simulink model "IARC_Nonlinear_Sensors"  (R2018a)
settings: Solver=ode1  StartTime=0.0  StopTime=20  FixedStep=T  RelTol=1e-3  EnableMultiTasking=on
undefined symbols (not defined in the file): A_1df, A_2df, alpha3, alpha_rp, alpha_x, alpha_z, an1, an1_v, an2, an3, bn1, bn1_v, bn2, bn3, dc_M_x, delta3, Epsilon3, F, g, Gamma1, Gamma2, Gamma3, Gamma4, gamma4_0, gamma_d_x, gamma_rp_0, gamma_x_0, gamma_z_0, Gammax, I, I_add, I_add_time, Jx, Jy, Jyaw, K, k1, k10, k11, k12, k2, k3, k4, k5, k6, k7, k8, k9, Ky, L, Light, LIMIT_CMD_PITCH, LIMIT_CMD_ROLL, LIMIT_CMD_xy, LIMIT_uCMD_HEIGHT, m, m_add, m_add_time, magnitude, MIL ... (+67)
libraries: simulink x131, simulink_extras x5, UAV_Control x4, aerolibwind2 x1
(part 3 of 6)

== system IARC_Nonlinear_Sensors/ARC Controller/Attitutde Control/Yaw control/e12 ==
  Add : Sum
  Discrete Derivative2 : simulink/Discrete/Discrete Derivative  gainval=1.0  ICPrevScaledInput=0.0  OutMin=[]  OutMax=[]  OutDataType=fixdt(1, 16)  OutScaling=2^-10  DoSatur=off
  Sum1 : Sum  Inputs=-+|
  Sum3 : Sum  Inputs=|+-
  Transfer Fcn3 : TransferFcn  Denominator=A_1df
  k11 : Gain  Gain=k11
  e12 : Outport
  wires:
  [psi_des] -> Sum3/2, Discrete Derivative2/1
  [psi] -> Sum3/1
  Sum1/1 -> Add/2  "ev"
  Sum3/1 -> k11/1  "ex"
  Add/1 -> e12/1
  [psi_dot] -> Sum1/2
  Discrete Derivative2/1 -> Transfer Fcn3/1
  k11/1 -> Add/1
  Transfer Fcn3/1 -> Sum1/1

== system IARC_Nonlinear_Sensors/ARC Controller/Attitutde Control/Yaw control/f ==
  " " : Trigonometry  Operator=sincos
  "  " : Trigonometry
  "      " : Trigonometry  Operator=cos
  Add : Sum  Inputs=++-
  Add1 : Sum  Inputs=+-
  Constant1 : Constant  Value=(Jy-Jyaw)/Jx
  Discrete Derivative1 : simulink/Discrete/Discrete Derivative  gainval=1.0  ICPrevScaledInput=0.0  OutMin=[]  OutMax=[]  OutDataType=fixdt(1, 16)  OutScaling=2^-10  DoSatur=off
  Discrete Derivative2 : simulink/Discrete/Discrete Derivative  gainval=1.0  ICPrevScaledInput=0.0  OutMin=[]  OutMax=[]  OutDataType=fixdt(1, 16)  OutScaling=2^-10  DoSatur=off
  Discrete Derivative3 : simulink/Discrete/Discrete Derivative  gainval=1.0  ICPrevScaledInput=0.0  OutMin=[]  OutMax=[]  OutDataType=fixdt(1, 16)  OutScaling=2^-10  DoSatur=off
  Ground : Ground
  Product1 : Product
  Product2 : Product  Inputs=**/
  Product4 : Product  Inputs=***/
  Selector1 : Selector  InputPortWidth=3  IndexOptions=Index vector (dialog)  Indices=[2 3]  OutputSizes=1
  q.r : Product  Inputs=*
  Out1 : Outport
  wires:
  [phi] -> "      "/1
  "      "/1 -> Product4/4
  Product4/1 -> Add/2
  q.r/1 -> Product4/2
  Selector1/1 -> q.r/1
  [pqr_est] -> Selector1/1
  Constant1/1 -> Product4/1
  Discrete Derivative1/1 -> Product2/1
  " "/2 -> Product2/3
  Add1/1 -> Product2/2
  Product1/1 -> Add1/2
  " "/1 -> Product1/2
  Discrete Derivative2/1 -> Product1/1
  Discrete Derivative3/1 -> Add1/1
  [phi] -> " "/1, Discrete Derivative1/1
  Add/1 -> Out1/1
  Product2/1 -> Add/1
  [theta] -> "  "/1
  "  "/1 -> Product4/3
  [psi] -> Discrete Derivative2/1
  [theta] -> Discrete Derivative3/1
  Ground/1 -> Add/3

== system IARC_Nonlinear_Sensors/ARC Controller/Attitutde Control/Yaw control/f(x) ==
  Add : Sum  Inputs=+--
  Discrete Derivative1 : simulink/Discrete/Discrete Derivative  gainval=1.0  ICPrevScaledInput=0.0  OutMin=[]  OutMax=[]  OutDataType=fixdt(1, 16)  OutScaling=2^-10  DoSatur=off
  T1 .. : Subsystem
  f : Subsystem
  Out1 : Outport
  wires:
  [psi_dot] -> Discrete Derivative1/1
  Discrete Derivative1/1 -> Add/1
  Add/1 -> Out1/1
  f/1(Out1) -> Add/2
  T1 ../1(Out1) -> Add/3

== system IARC_Nonlinear_Sensors/ARC Controller/Attitutde Control/Yaw control/phi ==
  "  " : Trigonometry  Operator=cos
  "   " : Trigonometry  Operator=cos
  Constant : Constant
  Gain10 : Gain  Gain=1/Ky
  Mux : Mux  Inputs=2
  Notch Filter2 : Subsystem
  Product2 : Product  Inputs=*/*
  rotor : TransferFcn  Numerator=1  Denominator=[Tm 1]
  Out1 : Outport
  wires:
  Mux/1 -> Out1/1
  Constant/1 -> Mux/2
  Notch Filter2/1(p) -> rotor/1
  [T3] -> Gain10/1
  "  "/1 -> Product2/1
  "   "/1 -> Product2/2
  rotor/1 -> Product2/3
  Product2/1 -> Mux/1
  [theta] -> "  "/1
  [phi] -> "   "/1
  Gain10/1 -> Notch Filter2/1(u)

== system IARC_Nonlinear_Sensors/ARC Controller/Attitutde Control/pitch control/Adaptation Law_X ==
  Phi_D : Inport
  error : Inport  Port=2
  f(x) : Inport  Port=3
  Phi_I : Inport  Port=4
  Adapt : Inport  Port=5
  " " : Subsystem
  Constant2 : Constant  Value=theta1_Max(1,2)
  Constant5 : Constant  Value=theta1_Max(1,1)
  Constant6 : Constant  Value=theta1_Min(1,2)
  Constant8 : Constant  Value=theta1_Min(1,1)
  Demux1 : Demux  Outputs=2
  Demux2 : Demux  Outputs=2
  Gain3 : Gain  Gain=K*L
  "IARC, Physical Model Based Parameter Estimation (69)_pitch (theta)" : Subsystem  AncestorBlock=|  mask(Physical Model Based Parameter Estimation){mu1=mu1_rp, mu2=mu2_rp, alpha=alpha_rp, nu=nu_rp, gamma0=gamma_rp_0, Rho_M=Rho_M_rp, Rho_L=Rho_L_rp, v=v_rp, theta_0=theta2_0, theta_max=theta2_Max, theta_min=theta2_Min, Theta_dot_M=theta_dot_M_rp, Tau=Tau_rp, t0=t0, Norm_ON=on}
      | UAV_Control/IARC, Physical Model Based 
      | Parameter Estimation (69)
      mask prompts: mu1 "forgetting factor, mu1:"; mu2 "RLS parameter, mu2:"; alpha "forgetting factor, alpha:"; nu "normalizing factor, nu:"; gamma0 "Initial adaptation gain:"; Rho_M "Upper bound for the adaptation gain:"; Rho_L "Lower bound for the adaptation gain:"; v "Eigenvector of Gamma_max:"; Theta_dot_M "Theta dot max:"; Tau "Filter time constant:"; t0 "Initialization Delay:"; Norm_ON "Use Normalized formula"
      mask Help:
      | Filtered system dynamics:
      | H_f (s)  is any stable LTI filter transfer function
      | x_f=H_f [x]
      | φ_f=H_f [φ(x)]
      | u_f=H_f [u]
      | 
      | y_p=x ̇_f−u_f
      | y ̂_p=φ_f^T θ ̂
      | Prediction error:
      | ϵ=y_p−y ̂_p
      | 
      | recursive estimation algorithms, the generalized parameter estimation algorithm (PAA) with covariance limiting:
      | 
      | θ ̂  ̇(t)=Γ(t) φ_f (t)ϵ(t)
      | D_Γ=μ_1 (t)Γ(t)−μ_2 (t)Γ(t) φ_f (t) φ_f (t)^T Γ(t)
      | Γ ̇(t)=D_Γ, if λ_M (Γ(t))<ρ_M  or v_M^T D_Γ v_M<0 )
      |          0        else
      | 
      | μ_1  and μ_2  are two non-negative functions
      | ρ_M  is a preset upper bound for the covariance matrix Γ(t)
      | μ_1  represents the forgetting factor (μ_1=0 for not forgetting)
      | μ_2: 1 stands for the standard least squares type estimation algorithm
      |        0 stands for  the gradient type estimation algorithm
      |        range: 0≤μ_2<2
      | Initialization of the covariance matrix: Γ(0)<ρ_M I_p
      | 
      | IARC designs completely separate the parameter estimation law design from the underlying robust control law to give better parameter estimates than possible with DARC designs. In addition, explicit on-line signal excitation level monitoring can be employed to significantly improve the accuracy of  parameter estimates.
      | 
      | Normalized Method:
      | θ ̂  ̇(t)=(Γ(t) φ_f (t)ϵ(t))/(1+νφ_f^T Γφ_f )
      | D_Γ=αΓ(t)−(Γ(t) φ_f (t) φ_f (t)^T Γ(t))/(1+νφ_f^T Γφ_f )
      | Γ ̇(t)=D_Γ, if λ_M (Γ(t))<ρ_M  or v_M^T D_Γ v_M<0
      |           0       else
      mask Display:
      | port_label('input',1,'f(x)','texmode','on')
      | port_label('input',2,'\phi','texmode','on')
      | port_label('input',3,'Adapt','texmode','on')
      | 
      | port_label('output',1,'\theta_{hat}','texmode','on')
  Integral Type Adaptation Law Discontinuous Projection1 : Subsystem  AncestorBlock=|  mask(IntegralTypeAdaptationLaw){theta=theta1, theta0=theta1_0, theta_max=theta1_Max, theta_min=theta1_Min, gamma=Gamma1, t0=t0, Adaptation_ON=on}
      | UAV_Control/Integral Type
      | Adaptation Law
      | Discontinuous Projection
      mask prompts: theta "Actual value of theta:"; theta0 "Initial value of theta:"; theta_max "Maximum value of theta:"; theta_min "Minimum value of theta:"; gamma "Adaptation Rate:"; t0 "Initialization Delay:"; Adaptation_ON "Activate adaptation:"
      mask help: Applies an Integral-type adaptation law with discontinuous projection on the parameter theta.
      mask Help:
      | Applies an Integral-type adaptation law with discontinuous projection on the parameter theta.
      | 
      | theta_est_dot=Gamma*Phi*e
      | theta=proj( int(theta_estdot) )
      | 
      | theta_min < theta_est <  theta_max
      | 
      | Parameters:
      | 
      | Gamma: nxn diagonal matrix, adaptaion rate.
      | theta_min: nx1 vector, minimum value of the estimated vector.
      | theta_max: nx1 vector, maximum value of the estimated vector.
      | theta0: nx1 vector, initial value of the estimated vector.
      | theta: nx1 vector, actual value of the estimated vector.
      | Adaptation_On: controls the use of the adaptation law (1: active, 0: inactive)
      | 
      | Inputs:
      | Phi: regressor vector, theta0, nx1.
      | e: state error, scalar.
      | 
      | Outputs:
      | theta_est: estimated value of the parameters vector.
      mask Display:
      | port_label('input',1,'\phi','texmode','on')
      | port_label('input',2,'e','texmode','on')
      | port_label('output',1,'\theta_{hat}','texmode','on')
  J : Subsystem
  Jyy : Scope
  KL/Jyy : Scope
  Manual Switch : ManualSwitch  CurrentSetting=0
  Manual Switch1 : ManualSwitch  CurrentSetting=0
  Math Function1 : Math  Operator=reciprocal  SaturateOnIntegerOverflow=on
  Mux1 : Mux  Inputs=5
  Mux6 : Mux  Inputs=5
  Subsystem1 : Subsystem
  To File : ToFile  Commented=on  Filename=IARC21.mat  MatrixName=IARC21  SaveFormat=Timeseries
  To File1 : ToFile  Commented=on  Filename=IARC22.mat  MatrixName=IARC22  SaveFormat=Timeseries
  To Workspace1 : ToWorkspace  Commented=on  VariableName=theta11  SaveFormat=Timeseries  SampleTime=-1
  To Workspace2 : ToWorkspace  Commented=on  VariableName=theta12  SaveFormat=Timeseries  SampleTime=-1
  d1 (N.m) : Scope
  theta1 : Outport
  theta2 : Outport  Port=2
  wires:
  " "/1(Out1) -> Mux6/3  "True"
  Gain3/1 -> To File/1, Jyy/1
  Constant2/1 -> Mux6/4
  Math Function1/1 -> Gain3/1
  Demux1/1 -> Manual Switch/2, KL/Jyy/1, Mux1/2
  Mux1/1 -> Math Function1/1
  Constant6/1 -> Mux6/5
  "IARC, Physical Model Based Parameter Estimation (69)_pitch (theta)"/1(Theta_hat) -> Demux1/1
  Demux2/1 -> Mux1/1, Manual Switch/1
  error/1 -> Integral Type Adaptation Law Discontinuous Projection1/2(error)
  Integral Type Adaptation Law Discontinuous Projection1/1(theta_est) -> Demux2/1
  Manual Switch1/1 -> To Workspace2/1, theta2/1
  J/1(Out1) -> Mux1/3
  Constant8/1 -> Mux1/5
  Phi_I/1 -> "IARC, Physical Model Based Parameter Estimation (69)_pitch (theta)"/2(Phi)
  f(x)/1 -> "IARC, Physical Model Based Parameter Estimation (69)_pitch (theta)"/1(f(x))
  Constant5/1 -> Mux1/4
  Manual Switch/1 -> To Workspace1/1, theta1/1
  Phi_D/1 -> Integral Type Adaptation Law Discontinuous Projection1/1(Phi)
  Mux6/1 -> Subsystem1/1(u)
  Demux2/2 -> Mux6/1, Manual Switch1/1
  Demux1/2 -> Mux6/2, Manual Switch1/2
  Subsystem1/1(y) -> To File1/1, d1 (N.m)/1
  Adapt/1 -> "IARC, Physical Model Based Parameter Estimation (69)_pitch (theta)"/3(Adapt)

== system IARC_Nonlinear_Sensors/ARC Controller/Attitutde Control/pitch control/Ix ==
  Constant : Constant
  Gain1 : Gain  Gain=L*K
  Product1 : Product  Inputs=*/
  " " : Outport
  wires:
  [theta11_est] -> Product1/2
  Gain1/1 -> " "/1
  Product1/1 -> Gain1/1
  Constant/1 -> Product1/1

== system IARC_Nonlinear_Sensors/ARC Controller/Attitutde Control/pitch control/Phi3 ==
  Constant : Constant
  Mux1 : Mux  Inputs=2
  Product1 : Product  Inputs=*/
  alpha 4 dot : Subsystem
  Out1 : Outport
  wires:
  Mux1/1 -> Out1/1
  Product1/1 -> Mux1/1
  Constant/1 -> Mux1/2
  alpha 4 dot/1(alpha_4_dot) -> Product1/1
  [theta11_est] -> Product1/2

== system IARC_Nonlinear_Sensors/ARC Controller/Attitutde Control/pitch control/Robust term ==
  e : Inport
  phi : Inport  Port=2
  Add : Sum
  Constant3 : Constant  Value=theta_max-theta_min
  Constant6 : Constant  Value=delta
  Gain : Gain  Gain=1/(4*epsilon)
  Math Function : Math  Operator=magnitude^2  SaturateOnIntegerOverflow=on
  Math Function1 : Math  Operator=magnitude^2  SaturateOnIntegerOverflow=on
  Math Function3 : Math  Operator=magnitude^2  SaturateOnIntegerOverflow=on
  Math Function5 : Math  Operator=transpose  SaturateOnIntegerOverflow=on
  Product : Product  Multiplication=Matrix(*)
  Product1 : Product
  alpha : Outport
  wires:
  phi/1 -> Math Function1/1
  e/1 -> Gain/1
  Math Function5/1 -> Product/1
  Product1/1 -> alpha/1
  Constant3/1 -> Math Function/1
  Math Function1/1 -> Math Function5/1
  Product/1 -> Add/1
  Math Function3/1 -> Add/2
  Constant6/1 -> Math Function3/1
  Math Function/1 -> Product/2
  Add/1 -> Product1/1
  Gain/1 -> Product1/2

== system IARC_Nonlinear_Sensors/ARC Controller/Attitutde Control/pitch control/T1 .. T2 .. ==
  "  " : Trigonometry  Operator=tan
  "    " : Trigonometry
  "     " : Trigonometry  Operator=cos
  "  2" : Trigonometry  Operator=tan
  Add : Sum  Inputs=+-
  Constant : Constant  Value=Jx
  Constant1 : Constant  Value=Jyaw
  Product1 : Product  Inputs=***/
  Product2 : Product  Inputs=***/
  Out1 : Outport
  wires:
  Constant/1 -> Product1/4
  [phi] -> "  "/1
  "  "/1 -> Product1/1
  [T1] -> Product1/3
  Product2/1 -> Add/2
  [theta] -> "    "/1
  "    "/1 -> Product1/2
  Add/1 -> Out1/1
  Product1/1 -> Add/1
  "     "/1 -> Product2/2
  [theta] -> "     "/1
  "  2"/1 -> Product2/1
  [phi] -> "  2"/1
  Constant1/1 -> Product2/4
  [T3] -> Product2/3

== system IARC_Nonlinear_Sensors/ARC Controller/Attitutde Control/pitch control/e4 ==
  Add : Sum
  Discrete Derivative2 : simulink/Discrete/Discrete Derivative  gainval=1.0  ICPrevScaledInput=0.0  OutMin=[]  OutMax=[]  OutDataType=fixdt(1, 16)  OutScaling=2^-10  DoSatur=off
  Sum1 : Sum  Inputs=-+|
  Sum3 : Sum  Inputs=|+-
  Transfer Fcn3 : TransferFcn  Denominator=A_1df
  k3 : Gain  Gain=k3
  e4 : Outport
  wires:
  Transfer Fcn3/1 -> Sum1/1
  k3/1 -> Add/1
  Discrete Derivative2/1 -> Transfer Fcn3/1
  [theta_dot] -> Sum1/2
  Add/1 -> e4/1
  Sum3/1 -> k3/1  "ex"
  Sum1/1 -> Add/2  "ev"
  [theta] -> Sum3/1
  [theta_d] -> Discrete Derivative2/1, Sum3/2

== system IARC_Nonlinear_Sensors/ARC Controller/Attitutde Control/pitch control/f(x) ==
  Add : Sum  Inputs=+--
  Discrete Derivative1 : simulink/Discrete/Discrete Derivative  gainval=1.0  ICPrevScaledInput=0.0  OutMin=[]  OutMax=[]  OutDataType=fixdt(1, 16)  OutScaling=2^-10  DoSatur=off
  T1 .. T3 .. : Subsystem
  f : Subsystem
  Out1 : Outport
  wires:
  T1 .. T3 ../1(Out1) -> Add/3
  f/1(Out1) -> Add/2
  Add/1 -> Out1/1
  Discrete Derivative1/1 -> Add/1
  [theta_dot] -> Discrete Derivative1/1

== system IARC_Nonlinear_Sensors/ARC Controller/Attitutde Control/pitch control/f1 ==
  " " : Trigonometry  Operator=sincos
  "  " : Trigonometry
  "      " : Trigonometry  Operator=tan
  Add : Sum  Inputs=+++-
  Add1 : Sum  Inputs=+-
  Constant : Constant  Value=(Jx-Jyaw)/Jy
  Constant1 : Constant  Value=(Jy-Jyaw)/Jx
  Discrete Derivative1 : simulink/Discrete/Discrete Derivative  gainval=1.0  ICPrevScaledInput=0.0  OutMin=[]  OutMax=[]  OutDataType=fixdt(1, 16)  OutScaling=2^-10  DoSatur=off
  Discrete Derivative2 : simulink/Discrete/Discrete Derivative  gainval=1.0  ICPrevScaledInput=0.0  OutMin=[]  OutMax=[]  OutDataType=fixdt(1, 16)  OutScaling=2^-10  DoSatur=off
  Discrete Derivative3 : simulink/Discrete/Discrete Derivative  gainval=1.0  ICPrevScaledInput=0.0  OutMin=[]  OutMax=[]  OutDataType=fixdt(1, 16)  OutScaling=2^-10  DoSatur=off
  Ground : Ground
  Product1 : Product
  Product2 : Product  Inputs=**/
  Product3 : Product
  Product4 : Product  Inputs=4
  Selector : Selector  InputPortWidth=3  IndexOptions=Index vector (dialog)  Indices=[1 3]  OutputSizes=1
  Selector1 : Selector  InputPortWidth=3  IndexOptions=Index vector (dialog)  Indices=[2 3]  OutputSizes=1
  p.r : Product  Inputs=*
  q.r : Product  Inputs=*
  Out1 : Outport
  wires:
  Ground/1 -> Add/3
  Product3/1 -> Add/2
  "  "/1 -> Product4/3
  [theta] -> "  "/1
  p.r/1 -> Product3/2
  Selector/1 -> p.r/1
  [pqr_est] -> Selector/1
  Constant/1 -> Product3/1
  Product2/1 -> Add/1
  Add/1 -> Out1/1
  [phi] -> Discrete Derivative1/1, " "/1
  Discrete Derivative3/1 -> Add1/1
  [psi] -> Discrete Derivative3/1
  [theta] -> Discrete Derivative2/1
  Discrete Derivative2/1 -> Product1/1
  " "/1 -> Product1/2
  Product1/1 -> Add1/2
  Add1/1 -> Product2/2
  " "/2 -> Product2/3
  Discrete Derivative1/1 -> Product2/1
  Constant1/1 -> Product4/1
  [pqr_est] -> Selector1/1
  Selector1/1 -> q.r/1
  q.r/1 -> Product4/2
  Product4/1 -> Add/4
  "      "/1 -> Product4/4
  [phi] -> "      "/1

== system IARC_Nonlinear_Sensors/ARC Controller/Attitutde Control/pitch control/phi ==
  Constant : Constant
  Gain10 : Gain  Gain=1/(L*K)
  Mux : Mux  Inputs=2
  Notch Filter2 : Subsystem
  rotor : TransferFcn  Numerator=1  Denominator=[Tm 1]
  Out1 : Outport
  wires:
  Notch Filter2/1(p) -> rotor/1
  rotor/1 -> Mux/1
  Constant/1 -> Mux/2
  Mux/1 -> Out1/1
  [T2] -> Gain10/1
  Gain10/1 -> Notch Filter2/1(u)

== system IARC_Nonlinear_Sensors/ARC Controller/Attitutde Control/roll control/Adaptation Law_Y ==
  Phi_D : Inport
  error : Inport  Port=2
  f(x) : Inport  Port=3
  Phi_I : Inport  Port=4
  Adapt : Inport  Port=5
  " " : Subsystem
  Constant2 : Constant  Value=theta2_Max(1,2)
  Constant5 : Constant  Value=theta2_Max(1,1)
  Constant6 : Constant  Value=theta2_Min(1,2)
  Constant8 : Constant  Value=theta2_Min(1,1)
  Demux1 : Demux  Outputs=2
  Demux2 : Demux  Outputs=2
  Gain3 : Gain  Gain=K*L
  "IARC, Physical Model Based Parameter Estimation (69)_roll (phi)" : Subsystem  AncestorBlock=|  mask(Physical Model Based Parameter Estimation){mu1=mu1_rp, mu2=mu2_rp, alpha=alpha_rp, nu=nu_rp, gamma0=gamma_rp_0, Rho_M=Rho_M_rp, Rho_L=Rho_L_rp, v=v_rp, theta_0=theta2_0, theta_max=theta2_Max, theta_min=theta2_Min, Theta_dot_M=theta_dot_M_rp, Tau=Tau_rp, t0=t0, Norm_ON=on}
      | UAV_Control/IARC, Physical Model Based 
      | Parameter Estimation (69)
      mask prompts: mu1 "forgetting factor, mu1:"; mu2 "RLS parameter, mu2:"; alpha "forgetting factor, alpha:"; nu "normalizing factor, nu:"; gamma0 "Initial adaptation gain:"; Rho_M "Upper bound for the adaptation gain:"; Rho_L "Lower bound for the adaptation gain:"; v "Eigenvector of Gamma_max:"; Theta_dot_M "Theta dot max:"; Tau "Filter time constant:"; t0 "Initialization Delay:"; Norm_ON "Use Normalized formula"
      mask Help:
      | Filtered system dynamics:
      | H_f (s)  is any stable LTI filter transfer function
      | x_f=H_f [x]
      | φ_f=H_f [φ(x)]
      | u_f=H_f [u]
      | 
      | y_p=x ̇_f−u_f
      | y ̂_p=φ_f^T θ ̂
      | Prediction error:
      | ϵ=y_p−y ̂_p
      | 
      | recursive estimation algorithms, the generalized parameter estimation algorithm (PAA) with covariance limiting:
      | 
      | θ ̂  ̇(t)=Γ(t) φ_f (t)ϵ(t)
      | D_Γ=μ_1 (t)Γ(t)−μ_2 (t)Γ(t) φ_f (t) φ_f (t)^T Γ(t)
      | Γ ̇(t)=D_Γ, if λ_M (Γ(t))<ρ_M  or v_M^T D_Γ v_M<0 )
      |          0        else
      | 
      | μ_1  and μ_2  are two non-negative functions
      | ρ_M  is a preset upper bound for the covariance matrix Γ(t)
      | μ_1  represents the forgetting factor (μ_1=0 for not forgetting)
      | μ_2: 1 stands for the standard least squares type estimation algorithm
      |        0 stands for  the gradient type estimation algorithm
      |        range: 0≤μ_2<2
      | Initialization of the covariance matrix: Γ(0)<ρ_M I_p
      | 
      | IARC designs completely separate the parameter estimation law design from the underlying robust control law to give better parameter estimates than possible with DARC designs. In addition, explicit on-line signal excitation level monitoring can be employed to significantly improve the accuracy of  parameter estimates.
      | 
      | Normalized Method:
      | θ ̂  ̇(t)=(Γ(t) φ_f (t)ϵ(t))/(1+νφ_f^T Γφ_f )
      | D_Γ=αΓ(t)−(Γ(t) φ_f (t) φ_f (t)^T Γ(t))/(1+νφ_f^T Γφ_f )
      | Γ ̇(t)=D_Γ, if λ_M (Γ(t))<ρ_M  or v_M^T D_Γ v_M<0
      |           0       else
      mask Display:
      | port_label('input',1,'f(x)','texmode','on')
      | port_label('input',2,'\phi','texmode','on')
      | port_label('input',3,'Adapt','texmode','on')
      | 
      | port_label('output',1,'\theta_{hat}','texmode','on')
  Integral Type Adaptation Law Discontinuous Projection : Subsystem  AncestorBlock=|  mask(IntegralTypeAdaptationLaw){theta=theta2, theta0=theta2_0, theta_max=theta2_Max, theta_min=theta2_Min, gamma=Gamma2, t0=t0, Adaptation_ON=on}
      | UAV_Control/Integral Type
      | Adaptation Law
      | Discontinuous Projection
      mask prompts: theta "Actual value of theta:"; theta0 "Initial value of theta:"; theta_max "Maximum value of theta:"; theta_min "Minimum value of theta:"; gamma "Adaptation Rate:"; t0 "Initialization Delay:"; Adaptation_ON "Activate adaptation:"
      mask help: Applies an Integral-type adaptation law with discontinuous projection on the parameter theta.
      mask Help:
      | Applies an Integral-type adaptation law with discontinuous projection on the parameter theta.
      | 
      | theta_est_dot=Gamma*Phi*e
      | theta=proj( int(theta_estdot) )
      | 
      | theta_min < theta_est <  theta_max
      | 
      | Parameters:
      | 
      | Gamma: nxn diagonal matrix, adaptaion rate.
      | theta_min: nx1 vector, minimum value of the estimated vector.
      | theta_max: nx1 vector, maximum value of the estimated vector.
      | theta0: nx1 vector, initial value of the estimated vector.
      | theta: nx1 vector, actual value of the estimated vector.
      | Adaptation_On: controls the use of the adaptation law (1: active, 0: inactive)
      | 
      | Inputs:
      | Phi: regressor vector, theta0, nx1.
      | e: state error, scalar.
      | 
      | Outputs:
      | theta_est: estimated value of the parameters vector.
      mask Display:
      | port_label('input',1,'\phi','texmode','on')
      | port_label('input',2,'e','texmode','on')
      | port_label('output',1,'\theta_{hat}','texmode','on')
  J : Subsystem
  Jxx : Scope
  KL/Jxx : Scope
  Manual Switch : ManualSwitch  CurrentSetting=0
  Manual Switch1 : ManualSwitch  CurrentSetting=0
  Math Function1 : Math  Operator=reciprocal  SaturateOnIntegerOverflow=on
  Mux1 : Mux  Inputs=5
  Mux6 : Mux  Inputs=5
  Subsystem2 : Subsystem
  To File : ToFile  Commented=on  Filename=IARC11.mat  MatrixName=IARC11  SaveFormat=Timeseries
  To File1 : ToFile  Commented=on  Filename=IARC12.mat  MatrixName=IARC12  SaveFormat=Timeseries
  To Workspace1 : ToWorkspace  Commented=on  VariableName=theta21  SaveFormat=Timeseries  SampleTime=-1
  To Workspace2 : ToWorkspace  Commented=on  VariableName=theta22  SaveFormat=Timeseries  SampleTime=-1
  d2(N.m) : Scope
  theta1 : Outport
  theta2 : Outport  Port=2
  wires:
  " "/1(Out1) -> Mux6/3
  Gain3/1 -> To File/1, Jxx/1
  Constant2/1 -> Mux6/4
  Math Function1/1 -> Gain3/1
  Demux1/1 -> Manual Switch/2, KL/Jxx/1, Mux1/2
  Mux1/1 -> Math Function1/1
  Constant6/1 -> Mux6/5
  "IARC, Physical Model Based Parameter Estimation (69)_roll (phi)"/1(Theta_hat) -> Demux1/1
  Demux2/1 -> Mux1/1, Manual Switch/1
  error/1 -> Integral Type Adaptation Law Discontinuous Projection/2(error)
  Integral Type Adaptation Law Discontinuous Projection/1(theta_est) -> Demux2/1
  J/1(Out1) -> Mux1/3
  Constant8/1 -> Mux1/5
  Phi_I/1 -> "IARC, Physical Model Based Parameter Estimation (69)_roll (phi)"/2(Phi)
  f(x)/1 -> "IARC, Physical Model Based Parameter Estimation (69)_roll (phi)"/1(f(x))
  Constant5/1 -> Mux1/4
  Phi_D/1 -> Integral Type Adaptation Law Discontinuous Projection/1(Phi)
  Mux6/1 -> Subsystem2/1(u)
  Demux2/2 -> Mux6/1, Manual Switch1/1
  Demux1/2 -> Mux6/2, Manual Switch1/2
  Adapt/1 -> "IARC, Physical Model Based Parameter Estimation (69)_roll (phi)"/3(Adapt)
  Manual Switch1/1 -> To Workspace2/1, theta2/1
  Manual Switch/1 -> To Workspace1/1, theta1/1
  Subsystem2/1(y) -> To File1/1, d2(N.m)/1

== system IARC_Nonlinear_Sensors/ARC Controller/Attitutde Control/roll control/Fast Dynamic Compensation Type Adaptation ==
  Z : Inport
  on : Inport  Port=2
  Divide : Product
  Gain : Gain  Gain=gamma_d
  Integrator : Integrator  LimitOutput=on  UpperSaturationLimit=dc_M  LowerSaturationLimit=-dc_M
  dc : Outport
  wires:
  Gain/1 -> Integrator/1
  Divide/1 -> Gain/1
  Integrator/1 -> dc/1
  Z/1 -> Divide/1
  on/1 -> Divide/2

== system IARC_Nonlinear_Sensors/ARC Controller/Attitutde Control/roll control/Phi3 ==
  Constant : Constant
  Mux1 : Mux  Inputs=2
  Product1 : Product  Inputs=*//
  alpha 8 dot : Subsystem
  cos : Trigonometry  Operator=cos
  Out1 : Outport
  wires:
  Constant/1 -> Mux1/2
  Product1/1 -> Mux1/1
  Mux1/1 -> Out1/1
  alpha 8 dot/1(alpha_8_dot) -> Product1/1
  cos/1 -> Product1/2
  [theta] -> cos/1
  [theta21_est] -> Product1/3

== system IARC_Nonlinear_Sensors/ARC Controller/Attitutde Control/roll control/Robust term ==
  e : Inport
  phi : Inport  Port=2
  Add : Sum
  Constant3 : Constant  Value=theta_max-theta_min
  Constant6 : Constant  Value=delta
  Gain : Gain  Gain=1/(4*epsilon)
  Math Function : Math  Operator=magnitude^2  SaturateOnIntegerOverflow=on
  Math Function1 : Math  Operator=magnitude^2  SaturateOnIntegerOverflow=on
  Math Function3 : Math  Operator=magnitude^2  SaturateOnIntegerOverflow=on
  Math Function5 : Math  Operator=transpose  SaturateOnIntegerOverflow=on
  Product : Product  Multiplication=Matrix(*)
  Product1 : Product
  alpha : Outport
  wires:
  Gain/1 -> Product1/2
  Add/1 -> Product1/1
  Math Function/1 -> Product/2
  Constant6/1 -> Math Function3/1
  Math Function3/1 -> Add/2
  Product/1 -> Add/1
  Math Function1/1 -> Math Function5/1
  Constant3/1 -> Math Function/1
  Product1/1 -> alpha/1
  Math Function5/1 -> Product/1
  e/1 -> Gain/1
  phi/1 -> Math Function1/1

== system IARC_Nonlinear_Sensors/ARC Controller/Attitutde Control/roll control/c_theta. Ix ==
  "  " : Trigonometry  Operator=cos
  Constant : Constant
  Gain1 : Gain  Gain=L*K
  Product1 : Product  Inputs=*//
  " " : Outport
  wires:
  [theta] -> "  "/1
  "  "/1 -> Product1/2
  Product1/1 -> Gain1/1
  Gain1/1 -> " "/1
  [theta21_est] -> Product1/3
  Constant/1 -> Product1/1

== system IARC_Nonlinear_Sensors/ARC Controller/Attitutde Control/roll control/e8 ==
  Add : Sum
  Discrete Derivative2 : simulink/Discrete/Discrete Derivative  gainval=1.0  ICPrevScaledInput=0.0  OutMin=[]  OutMax=[]  OutDataType=fixdt(1, 16)  OutScaling=2^-10  DoSatur=off
  Sum1 : Sum  Inputs=-+|
  Sum3 : Sum  Inputs=|+-
  Transfer Fcn3 : TransferFcn  Denominator=A_1df
  k7 : Gain  Gain=k7
  e8 : Outport
  wires:
  [phi_d] -> Sum3/2, Discrete Derivative2/1
  [phi] -> Sum3/1
  Sum1/1 -> Add/2  "ev"
  Sum3/1 -> k7/1  "ex"
  Add/1 -> e8/1
  [phi_dot] -> Sum1/2
  Discrete Derivative2/1 -> Transfer Fcn3/1
  k7/1 -> Add/1
  Transfer Fcn3/1 -> Sum1/1

== system IARC_Nonlinear_Sensors/ARC Controller/Attitutde Control/roll control/f ==
  " " : Trigonometry  Operator=cos
  "  " : Trigonometry
  Add : Sum  Inputs=---
  Constant : Constant  Value=(Jy-Jyaw)/Jx
  Discrete Derivative2 : simulink/Discrete/Discrete Derivative  gainval=1.0  ICPrevScaledInput=0.0  OutMin=[]  OutMax=[]  OutDataType=fixdt(1, 16)  OutScaling=2^-10  DoSatur=off
  Discrete Derivative3 : simulink/Discrete/Discrete Derivative  gainval=1.0  ICPrevScaledInput=0.0  OutMin=[]  OutMax=[]  OutDataType=fixdt(1, 16)  OutScaling=2^-10  DoSatur=off
  Ground : Ground
  Product2 : Product  Inputs=3
  Product3 : Product  Inputs=3
  Selector : Selector  InputPortWidth=3  IndexOptions=Index vector (dialog)  Indices=[2 3]  OutputSizes=1
  q.r : Product  Inputs=*
  Out1 : Outport
  wires:
  [theta] -> Discrete Derivative2/1
  [psi] -> Discrete Derivative3/1
  Discrete Derivative2/1 -> Product2/1
  Discrete Derivative3/1 -> Product2/2
  [phi] -> " "/1
  " "/1 -> Product2/3
  Add/1 -> Out1/1
  Product2/1 -> Add/1
  Constant/1 -> Product3/1
  [pqr_est] -> Selector/1
  Selector/1 -> q.r/1
  q.r/1 -> Product3/2
  [theta] -> "  "/1
  "  "/1 -> Product3/3
  Product3/1 -> Add/2
  Ground/1 -> Add/3

== system IARC_Nonlinear_Sensors/ARC Controller/Attitutde Control/roll control/f(x) ==
  Add : Sum  Inputs=+--
  Discrete Derivative1 : simulink/Discrete/Discrete Derivative  gainval=1.0  ICPrevScaledInput=0.0  OutMin=[]  OutMax=[]  OutDataType=fixdt(1, 16)  OutScaling=2^-10  DoSatur=off
  f : Subsystem
  s_theta.T3/Iz : Subsystem
  Out1 : Outport
  wires:
  [phi_dot] -> Discrete Derivative1/1
  Discrete Derivative1/1 -> Add/1
  Add/1 -> Out1/1
  f/1(Out1) -> Add/2
  s_theta.T3/Iz/1(Out1) -> Add/3

== system IARC_Nonlinear_Sensors/ARC Controller/Attitutde Control/roll control/phi ==
  "  " : Trigonometry  Operator=cos
  Constant : Constant
  Gain10 : Gain  Gain=1/(L*K)
  Mux : Mux  Inputs=2
  Notch Filter2 : Subsystem
  c_theta . T1 : Product
  rotor : TransferFcn  Numerator=1  Denominator=[Tm 1]
  Out1 : Outport
  wires:
  Mux/1 -> Out1/1
  "  "/1 -> c_theta . T1/1
  [theta] -> "  "/1
  Constant/1 -> Mux/2
  c_theta . T1/1 -> Mux/1
  Notch Filter2/1(p) -> rotor/1
  rotor/1 -> c_theta . T1/2
  [T1] -> Gain10/1
  Gain10/1 -> Notch Filter2/1(u)

== system IARC_Nonlinear_Sensors/ARC Controller/Attitutde Control/roll control/s_theta.T3//Iz ==
  "  " : Trigonometry
  Constant : Constant  Value=Jyaw
  Product1 : Product  Inputs=**/
  Out1 : Outport
  wires:
  "  "/1 -> Product1/1
  [theta] -> "  "/1
  Constant/1 -> Product1/3
  Product1/1 -> Out1/1
  [T3] -> Product1/2

== system IARC_Nonlinear_Sensors/ARC Controller/Position Control/Coupling/Warm Up+Sat ==
  In1 : Inport
  Mux : Mux  Inputs=2
  Saturation : Saturate  UpperLimit=2*LIMIT_uCMD_HEIGHT  LowerLimit=0.7*LIMIT_uCMD_HEIGHT
  Scope1 : Scope
  Scope2 : Scope
  Scope3 : Scope
  Warm Up : Subsystem
  u1 (N) : Outport
  tag scope: Adapt_M=global, takeoff=global
  wires:
  Saturation/1 -> Mux/1, Warm Up/1(u)
  [z] -> Warm Up/2(z)
  Warm Up/3(Adapt_J) -> Scope2/1, [takeoff]
  Warm Up/1(y) -> Mux/2, u1 (N)/1
  Warm Up/2(Adapt_M) -> Scope1/1, [Adapt_M]
  In1/1 -> Saturation/1
  [z_des] -> Warm Up/3(z_des)
  Mux/1 -> Scope3/1

== system IARC_Nonlinear_Sensors/ARC Controller/Position Control/Coupling/x m_hat ==
  " " : Inport
  "  " : Product
  Constant : Constant  Value=K
  m_hat : Product  Inputs=*/
  u1_des (N) : Outport
  wires:
  Constant/1 -> m_hat/1
  m_hat/1 -> "  "/1
  "  "/1 -> u1_des (N)/1
  [theta31_est] -> m_hat/2
  " "/1 -> "  "/2

== system IARC_Nonlinear_Sensors/ARC Controller/Position Control/X control/Adaptation Law_X ==
  f(x) : Inport
  Phi_I : Inport  Port=2
  Adapt : Inport  Port=3
  Phi_d : Inport  Port=4
  error : Inport  Port=5
  " " : Subsystem
  (N) : Scope
  Constant2 : Constant  Value=thetax_Max
  Constant6 : Constant  Value=thetax_Min
  "IARC, Physical Model Based Parameter Estimation (69)_X" : Subsystem  AncestorBlock=|  mask(Physical Model Based Parameter Estimation){mu1=mu1_x, mu2=mu2_x, alpha=alpha_x, nu=nu_x, gamma0=gamma_x_0, Rho_M=Rho_M_x, Rho_L=Rho_L_x, v=v_x, theta_0=thetax_0, theta_max=thetax_Max, theta_min=thetax_Min, Theta_dot_M=theta_dot_M_x, Tau=Tau_x, t0=t0, Norm_ON=on}
      | UAV_Control/IARC, Physical Model Based 
      | Parameter Estimation (69)
      mask prompts: mu1 "forgetting factor, mu1:"; mu2 "RLS parameter, mu2:"; alpha "forgetting factor, alpha:"; nu "normalizing factor, nu:"; gamma0 "Initial adaptation gain:"; Rho_M "Upper bound for the adaptation gain:"; Rho_L "Lower bound for the adaptation gain:"; v "Eigenvector of Gamma_max:"; Theta_dot_M "Theta dot max:"; Tau "Filter time constant:"; t0 "Initialization Delay:"; Norm_ON "Use Normalized formula"
      mask Help:
      | Filtered system dynamics:
      | H_f (s)  is any stable LTI filter transfer function
      | x_f=H_f [x]
      | φ_f=H_f [φ(x)]
      | u_f=H_f [u]
      | 
      | y_p=x ̇_f−u_f
      | y ̂_p=φ_f^T θ ̂
      | Prediction error:
      | ϵ=y_p−y ̂_p
      | 
      | recursive estimation algorithms, the generalized parameter estimation algorithm (PAA) with covariance limiting:
      | 
      | θ ̂  ̇(t)=Γ(t) φ_f (t)ϵ(t)
      | D_Γ=μ_1 (t)Γ(t)−μ_2 (t)Γ(t) φ_f (t) φ_f (t)^T Γ(t)
      | Γ ̇(t)=D_Γ, if λ_M (Γ(t))<ρ_M  or v_M^T D_Γ v_M<0 )
      |          0        else
      | 
      | μ_1  and μ_2  are two non-negative functions
      | ρ_M  is a preset upper bound for the covariance matrix Γ(t)
      | μ_1  represents the forgetting factor (μ_1=0 for not forgetting)
      | μ_2: 1 stands for the standard least squares type estimation algorithm
      |        0 stands for  the gradient type estimation algorithm
      |        range: 0≤μ_2<2
      | Initialization of the covariance matrix: Γ(0)<ρ_M I_p
      | 
      | IARC designs completely separate the parameter estimation law design from the underlying robust control law to give better parameter estimates than possible with DARC designs. In addition, explicit on-line signal excitation level monitoring can be employed to significantly improve the accuracy of  parameter estimates.
      | 
      | Normalized Method:
      | θ ̂  ̇(t)=(Γ(t) φ_f (t)ϵ(t))/(1+νφ_f^T Γφ_f )
      | D_Γ=αΓ(t)−(Γ(t) φ_f (t) φ_f (t)^T Γ(t))/(1+νφ_f^T Γφ_f )
      | Γ ̇(t)=D_Γ, if λ_M (Γ(t))<ρ_M  or v_M^T D_Γ v_M<0
      |           0       else
      mask Display:
      | port_label('input',1,'f(x)','texmode','on')
      | port_label('input',2,'\phi','texmode','on')
      | port_label('input',3,'Adapt','texmode','on')
      | 
      | port_label('output',1,'\theta_{hat}','texmode','on')
  Integral Type Adaptation Law Discontinuous Projection1 : Subsystem  AncestorBlock=|  mask(IntegralTypeAdaptationLaw){theta=thetax, theta0=thetax_0, theta_max=thetax_Max, theta_min=thetax_Min, gamma=Gammax, t0=3, Adaptation_ON=on}
      | UAV_Control/Integral Type
      | Adaptation Law
      | Discontinuous Projection
      mask prompts: theta "Actual value of theta:"; theta0 "Initial value of theta:"; theta_max "Maximum value of theta:"; theta_min "Minimum value of theta:"; gamma "Adaptation Rate:"; t0 "Initialization Delay:"; Adaptation_ON "Activate adaptation:"
      mask help: Applies an Integral-type adaptation law with discontinuous projection on the parameter theta.
      mask Help:
      | Applies an Integral-type adaptation law with discontinuous projection on the parameter theta.
      | 
      | theta_est_dot=Gamma*Phi*e
      | theta=proj( int(theta_estdot) )
      | 
      | theta_min < theta_est <  theta_max
      | 
      | Parameters:
      | 
      | Gamma: nxn diagonal matrix, adaptaion rate.
      | theta_min: nx1 vector, minimum value of the estimated vector.
      | theta_max: nx1 vector, maximum value of the estimated vector.
      | theta0: nx1 vector, initial value of the estimated vector.
      | theta: nx1 vector, actual value of the estimated vector.
      | Adaptation_On: controls the use of the adaptation law (1: active, 0: inactive)
      | 
      | Inputs:
      | Phi: regressor vector, theta0, nx1.
      | e: state error, scalar.
      | 
      | Outputs:
      | theta_est: estimated value of the parameters vector.
      mask Display:
      | port_label('input',1,'\phi','texmode','on')
      | port_label('input',2,'e','texmode','on')
      | port_label('output',1,'\theta_{hat}','texmode','on')
  Manual Switch : ManualSwitch
  Mux6 : Mux  Inputs=5
  Subsystem1 : Subsystem
  dx : Scope
  theta1 : Outport
  wires:
  " "/1(Out1) -> Mux6/3  "True"
  Phi_I/1 -> "IARC, Physical Model Based Parameter Estimation (69)_X"/2(Phi)
  f(x)/1 -> "IARC, Physical Model Based Parameter Estimation (69)_X"/1(f(x))
  Mux6/1 -> Subsystem1/1(u)
  Subsystem1/1(y) -> (N)/1
  Adapt/1 -> "IARC, Physical Model Based Parameter Estimation (69)_X"/3(Adapt)
  "IARC, Physical Model Based Parameter Estimation (69)_X"/1(Theta_hat) -> dx/1, Mux6/2, Manual Switch/2
  Constant2/1 -> Mux6/4
  Constant6/1 -> Mux6/5
  Phi_d/1 -> Integral Type Adaptation Law Discontinuous Projection1/1(Phi)
  error/1 -> Integral Type Adaptation Law Discontinuous Projection1/2(error)
  Integral Type Adaptation Law Discontinuous Projection1/1(theta_est) -> Mux6/1, Manual Switch/1
  Manual Switch/1 -> theta1/1

== system IARC_Nonlinear_Sensors/ARC Controller/Position Control/X control/Fast Dynamic Compensation Type Adaptation ==
  Z : Inport
  on : Inport  Port=2
  Divide : Product
  Gain : Gain  Gain=gamma_d
  Integrator : Integrator  LimitOutput=on  UpperSaturationLimit=dc_M  LowerSaturationLimit=-dc_M
  dc : Outport
  wires:
  Gain/1 -> Integrator/1
  Divide/1 -> Gain/1
  Integrator/1 -> dc/1
  Z/1 -> Divide/1
  on/1 -> Divide/2

== system IARC_Nonlinear_Sensors/ARC Controller/Position Control/X control/e2 ==
  Add : Sum
  Discrete Derivative2 : simulink/Discrete/Discrete Derivative  gainval=1.0  ICPrevScaledInput=0.0  OutMin=[]  OutMax=[]  OutDataType=fixdt(1, 16)  OutScaling=2^-10  DoSatur=off
  Sum1 : Sum  Inputs=-+|
  Sum3 : Sum  Inputs=|+-
  k1 : Gain  Gain=k1
  e2 : Outport
  wires:
  [x_des] -> Sum3/2, Discrete Derivative2/1
  [x] -> Sum3/1
  Sum1/1 -> Add/2  "ev"
  Sum3/1 -> k1/1  "ex"
  Add/1 -> e2/1
  [x_dot] -> Sum1/2
  Discrete Derivative2/1 -> Sum1/1
  k1/1 -> Add/1

== system IARC_Nonlinear_Sensors/ARC Controller/Position Control/X control/f(x) ==
  "  " : Gain  Gain=1/m
  Discrete Derivative1 : simulink/Discrete/Discrete Derivative  gainval=1.0  ICPrevScaledInput=0.0  OutMin=[]  OutMax=[]  OutDataType=fixdt(1, 16)  OutScaling=2^-10  DoSatur=off
  Fcn13 : Fcn  Expr=u(1)*u(5)*u(3) + u(2)*u(6)
  Mux : Mux  Inputs=2
  Mux2 : Mux  Inputs=3
  Product1 : Product
  Sum2 : Sum  Inputs=|+-
  rotor2 : TransferFcn  Numerator=1  Denominator=[Tm 1]
  sincos : Trigonometry  Operator=sincos
  Out1 : Outport
  wires:
  sincos/2 -> Mux/2
  [x_dot] -> Discrete Derivative1/1
  [theta] -> Mux2/2
  Product1/1 -> Sum2/2
  [phi] -> Mux2/1
  [psi] -> Mux2/3
  Discrete Derivative1/1 -> Sum2/1
  Mux/1 -> Fcn13/1
  sincos/1 -> Mux/1
  Mux2/1 -> sincos/1
  Fcn13/1 -> Product1/1
  [Fz_des] -> "  "/1
  Sum2/1 -> Out1/1
  rotor2/1 -> Product1/2
  "  "/1 -> rotor2/1

== system IARC_Nonlinear_Sensors/ARC Controller/Position Control/Y control/Adaptation Law_Y ==
  f(x) : Inport
  Phi_I : Inport  Port=2
  Adapt : Inport  Port=3
  Phi_d : Inport  Port=4
  error : Inport  Port=5
  " " : Subsystem
  (N) : Scope
  Constant2 : Constant  Value=thetax_Max
  Constant6 : Constant  Value=thetax_Min
  "IARC, Physical Model Based Parameter Estimation (69)_X" : Subsystem  AncestorBlock=|  mask(Physical Model Based Parameter Estimation){mu1=mu1_x, mu2=mu2_x, alpha=alpha_x, nu=nu_x, gamma0=gamma_x_0, Rho_M=Rho_M_x, Rho_L=Rho_L_x, v=v_x, theta_0=thetax_0, theta_max=thetax_Max, theta_min=thetax_Min, Theta_dot_M=theta_dot_M_x, Tau=Tau_x, t0=t0, Norm_ON=on}
      | UAV_Control/IARC, Physical Model Based 
      | Parameter Estimation (69)
      mask prompts: mu1 "forgetting factor, mu1:"; mu2 "RLS parameter, mu2:"; alpha "forgetting factor, alpha:"; nu "normalizing factor, nu:"; gamma0 "Initial adaptation gain:"; Rho_M "Upper bound for the adaptation gain:"; Rho_L "Lower bound for the adaptation gain:"; v "Eigenvector of Gamma_max:"; Theta_dot_M "Theta dot max:"; Tau "Filter time constant:"; t0 "Initialization Delay:"; Norm_ON "Use Normalized formula"
      mask Help:
      | Filtered system dynamics:
      | H_f (s)  is any stable LTI filter transfer function
      | x_f=H_f [x]
      | φ_f=H_f [φ(x)]
      | u_f=H_f [u]
      | 
      | y_p=x ̇_f−u_f
      | y ̂_p=φ_f^T θ ̂
      | Prediction error:
      | ϵ=y_p−y ̂_p
      | 
      | recursive estimation algorithms, the generalized parameter estimation algorithm (PAA) with covariance limiting:
      | 
      | θ ̂  ̇(t)=Γ(t) φ_f (t)ϵ(t)
      | D_Γ=μ_1 (t)Γ(t)−μ_2 (t)Γ(t) φ_f (t) φ_f (t)^T Γ(t)
      | Γ ̇(t)=D_Γ, if λ_M (Γ(t))<ρ_M  or v_M^T D_Γ v_M<0 )
      |          0        else
      | 
      | μ_1  and μ_2  are two non-negative functions
      | ρ_M  is a preset upper bound for the covariance matrix Γ(t)
      | μ_1  represents the forgetting factor (μ_1=0 for not forgetting)
      | μ_2: 1 stands for the standard least squares type estimation algorithm
      |        0 stands for  the gradient type estimation algorithm
      |        range: 0≤μ_2<2
      | Initialization of the covariance matrix: Γ(0)<ρ_M I_p
      | 
      | IARC designs completely separate the parameter estimation law design from the underlying robust control law to give better parameter estimates than possible with DARC designs. In addition, explicit on-line signal excitation level monitoring can be employed to significantly improve the accuracy of  parameter estimates.
      | 
      | Normalized Method:
      | θ ̂  ̇(t)=(Γ(t) φ_f (t)ϵ(t))/(1+νφ_f^T Γφ_f )
      | D_Γ=αΓ(t)−(Γ(t) φ_f (t) φ_f (t)^T Γ(t))/(1+νφ_f^T Γφ_f )
      | Γ ̇(t)=D_Γ, if λ_M (Γ(t))<ρ_M  or v_M^T D_Γ v_M<0
      |           0       else
      mask Display:
      | port_label('input',1,'f(x)','texmode','on')
      | port_label('input',2,'\phi','texmode','on')
      | port_label('input',3,'Adapt','texmode','on')
      | 
      | port_label('output',1,'\theta_{hat}','texmode','on')
  Integral Type Adaptation Law Discontinuous Projection1 : Subsystem  AncestorBlock=|  mask(IntegralTypeAdaptationLaw){theta=thetax, theta0=thetax_0, theta_max=thetax_Max, theta_min=thetax_Min, gamma=Gammax, t0=3, Adaptation_ON=on}
      | UAV_Control/Integral Type
      | Adaptation Law
      | Discontinuous Projection
      mask prompts: theta "Actual value of theta:"; theta0 "Initial value of theta:"; theta_max "Maximum value of theta:"; theta_min "Minimum value of theta:"; gamma "Adaptation Rate:"; t0 "Initialization Delay:"; Adaptation_ON "Activate adaptation:"
      mask help: Applies an Integral-type adaptation law with discontinuous projection on the parameter theta.
      mask Help:
      | Applies an Integral-type adaptation law with discontinuous projection on the parameter theta.
      | 
      | theta_est_dot=Gamma*Phi*e
      | theta=proj( int(theta_estdot) )
      | 
      | theta_min < theta_est <  theta_max
      | 
      | Parameters:
      | 
      | Gamma: nxn diagonal matrix, adaptaion rate.
      | theta_min: nx1 vector, minimum value of the estimated vector.
      | theta_max: nx1 vector, maximum value of the estimated vector.
      | theta0: nx1 vector, initial value of the estimated vector.
      | theta: nx1 vector, actual value of the estimated vector.
      | Adaptation_On: controls the use of the adaptation law (1: active, 0: inactive)
      | 
      | Inputs:
      | Phi: regressor vector, theta0, nx1.
      | e: state error, scalar.
      | 
      | Outputs:
      | theta_est: estimated value of the parameters vector.
      mask Display:
      | port_label('input',1,'\phi','texmode','on')
      | port_label('input',2,'e','texmode','on')
      | port_label('output',1,'\theta_{hat}','texmode','on')
  Manual Switch : ManualSwitch
  Mux6 : Mux  Inputs=5
  Subsystem1 : Subsystem
  dx : Scope
  theta1 : Outport
  wires:
  " "/1(Out1) -> Mux6/3  "True"
  Phi_I/1 -> "IARC, Physical Model Based Parameter Estimation (69)_X"/2(Phi)
  f(x)/1 -> "IARC, Physical Model Based Parameter Estimation (69)_X"/1(f(x))
  Mux6/1 -> Subsystem1/1(u)
  Subsystem1/1(y) -> (N)/1
  Adapt/1 -> "IARC, Physical Model Based Parameter Estimation (69)_X"/3(Adapt)
  "IARC, Physical Model Based Parameter Estimation (69)_X"/1(Theta_hat) -> dx/1, Mux6/2, Manual Switch/2
  Constant2/1 -> Mux6/4
  Constant6/1 -> Mux6/5
  Phi_d/1 -> Integral Type Adaptation Law Discontinuous Projection1/1(Phi)
  error/1 -> Integral Type Adaptation Law Discontinuous Projection1/2(error)
  Integral Type Adaptation Law Discontinuous Projection1/1(theta_est) -> Mux6/1, Manual Switch/1
  Manual Switch/1 -> theta1/1

== system IARC_Nonlinear_Sensors/ARC Controller/Position Control/Y control/Fast Dynamic Compensation Type Adaptation ==
  Z : Inport
  on : Inport  Port=2
  Divide : Product
  Gain : Gain  Gain=gamma_d
  Integrator : Integrator  LimitOutput=on  UpperSaturationLimit=dc_M  LowerSaturationLimit=-dc_M
  dc : Outport
  wires:
  Gain/1 -> Integrator/1
  Divide/1 -> Gain/1
  Integrator/1 -> dc/1
  Z/1 -> Divide/1
  on/1 -> Divide/2

== system IARC_Nonlinear_Sensors/ARC Controller/Position Control/Y control/e2 ==
  Add : Sum
  Discrete Derivative2 : simulink/Discrete/Discrete Derivative  gainval=1.0  ICPrevScaledInput=0.0  OutMin=[]  OutMax=[]  OutDataType=fixdt(1, 16)  OutScaling=2^-10  DoSatur=off
  Sum1 : Sum  Inputs=-+|
  Sum3 : Sum  Inputs=|+-
  k1 : Gain  Gain=k5
  e6 : Outport
  wires:
  [y_des] -> Sum3/2, Discrete Derivative2/1
  [y] -> Sum3/1
  Sum1/1 -> Add/2  "ev"
  Sum3/1 -> k1/1  "ex"
  Add/1 -> e6/1
  [y_dot] -> Sum1/2
  Discrete Derivative2/1 -> Sum1/1
  k1/1 -> Add/1

== system IARC_Nonlinear_Sensors/ARC Controller/Position Control/Y control/f(x)1 ==
  "  " : Gain  Gain=1/m
  Discrete Derivative1 : simulink/Discrete/Discrete Derivative  gainval=1.0  ICPrevScaledInput=0.0  OutMin=[]  OutMax=[]  OutDataType=fixdt(1, 16)  OutScaling=2^-10  DoSatur=off
  Fcn23 : Fcn  Expr=-u(1)*u(5)*u(6) + u(2)*u(3)
  Mux : Mux  Inputs=2
  Mux2 : Mux  Inputs=3
  Product1 : Product
  Sum2 : Sum  Inputs=|+-
  rotor2 : TransferFcn  Numerator=1  Denominator=[Tm 1]
  sincos : Trigonometry  Operator=sincos
  Out1 : Outport
  wires:
  rotor2/1 -> Product1/2
  Sum2/1 -> Out1/1
  [Fz_des] -> "  "/1
  Fcn23/1 -> Product1/1
  Mux2/1 -> sincos/1
  sincos/1 -> Mux/1
  Mux/1 -> Fcn23/1
  Discrete Derivative1/1 -> Sum2/1
  [psi] -> Mux2/3
  [phi] -> Mux2/1
  Product1/1 -> Sum2/2
  [theta] -> Mux2/2
  [y_dot] -> Discrete Derivative1/1
  sincos/2 -> Mux/2
  "  "/1 -> rotor2/1

== system IARC_Nonlinear_Sensors/ARC Controller/Position Control/Z control/ARC block ==
  e : Inport
  phi : Inport  Port=2
  Add : Sum
  Constant3 : Constant  Value=theta_max-theta_min
  Constant6 : Constant  Value=delta
  Gain : Gain  Gain=1/(4*epsilon)
  Math Function : Math  Operator=magnitude^2  SaturateOnIntegerOverflow=on
  Math Function1 : Math  Operator=magnitude^2  SaturateOnIntegerOverflow=on
  Math Function3 : Math  Operator=magnitude^2  SaturateOnIntegerOverflow=on
  Math Function5 : Math  Operator=transpose  SaturateOnIntegerOverflow=on
  Product : Product  Multiplication=Matrix(*)
  Product1 : Product
  alpha : Outport
  wires:
  Gain/1 -> Product1/2
  Add/1 -> Product1/1
  Math Function/1 -> Product/2
  Constant6/1 -> Math Function3/1
  Math Function3/1 -> Add/2
  Product/1 -> Add/1
  Math Function1/1 -> Math Function5/1
  Constant3/1 -> Math Function/1
  Product1/1 -> alpha/1
  Math Function5/1 -> Product/1
  e/1 -> Gain/1
  phi/1 -> Math Function1/1
